simulink model "OUR_BD_FUELCELL"  (R2022b)
settings: Solver=ode1  StartTime=0.0  StopTime=max(cyc_mph(:,1))  FixedStep=1  MaxStep=1  RelTol=1e-3  AbsTol=1e-3
values from neighbouring files (symbols this model uses):
  eta_DC_DC = 1    [main.m]
  fc_pwr_scale = 0.6    [fuelcell_patch.m]
  Ts = 1    [main.m]
undefined symbols (not defined in the file or in its folder): air_cp, amb_tmp, cs_charge_deplete_bool, cs_charge_pwr, cs_fc_init_state, cs_fc_on, cs_hi_soc, cs_lo_soc, cs_max_pwr, cs_max_pwr_fall_rate, cs_max_pwr_rise_rate, cs_min_off_time, cs_min_pwr, ess_on, ex_calc, ex_gas_cp, fc_acc_mass, fc_base_mass, fc_c2i_th_cond, fc_c_init_tmp, fc_cl2h_eff, fc_co_map, fc_co_map_c2h, fc_cold, fc_cold_tmp, fc_cp, fc_eff_scale, fc_emis, fc_emisv, fc_exflow_map, fc_ext_sarea, fc_extmp_map, fc_fuel_den, fc_fuel_lhv, fc_fuel_map, fc_fuel_map_c2h, fc_fuelcell_warmup_bool, fc_h2x_th_cond, fc_h_air_flow, fc_h_cp, fc_h_init_tmp, fc_hc_map, fc_hc_map_c2h, fc_hood_emisv, fc_hood_sarea, fc_i2x_th_cond, fc_i_init_tmp, fc_nox_map, fc_nox_map_c2h, fc_o2_map, fc_on, fc_pm_map, fc_pm_map_c2h, fc_pwr_map, fc_tstat, fc_x_init_tmp, pow, veh_glider_mass
libraries: lib_wheel x2, lib_help x2, lib_transmission x2, lib_outputs x1, lib_controls x1, lib_interactive x1, lib_drive_cycle x1, lib_accessory x1, lib_energy_storage x1, lib_exhaust x1, mpclib x1, lib_electric_machine x1
(part 1 of 2)
settings Model: ModifiedComment=utente -- Tue Jun 25 17:18:19 2024 -- Version 21.0  Creator=mokeefe  LastModifiedBy=William
settings Model: ModifiedHistory=|
  | utente -- Tue Jun 25 17:18:19 2024 -- Version 21.0
  | 
  | mokeefe -- Fri Mar 23 15:51:49 2012 -- Version 1.79
  | Upgrade parameterized links and upgrade file to latest Simulink.
  | 
  | ssprik -- Wed Sep 24 14:55:17 2003 -- Version 1.78
  | 
  | 
  | kharalds -- Tue Jun 10 10:04:01 2003 -- Version 1.77
  | undid the prior change (back to 10000) in Fuel Cell Power System Model/min_cell_voltage & net power gen/algebraic constraint/initial guess
  | 
  | kharalds -- Tue Jun 10 09:48:54 2003 -- Version 1.76
  | in Fuel Cell Power System Model/min_cell_voltage & net power gen/algebraic constraint/Initial guess: changed value from 40000 to 10000.
  | 
  | bjeanner -- Tue Dec 10 15:48:38 2002 -- Version 1.75
  | 
  | 
  | bjeanner -- Tue Dec 10 15:20:32 2002 -- Version 1.74
  | 
  | 
  | bjeanner -- Tue Dec 10 11:52:09 2002 -- Version 1.73
  | 
  | 
  | bjeanner -- Tue Dec 10 11:30:33 2002 -- Version 1.72
  | 
  | 
  | bjeanner -- Tue Dec 10 11:22:18 2002 -- Version 1.71
  | 
  | 
  | bjeanner -- Tue Dec 10 11:18:18 2002 -- Version 1.70
  | 
  | 
  | bjeanner -- Tue Dec 10 10:31:06 2002 -- Version 1.69
  | 
  | 
  | bjeanner -- Tue Dec 10 10:30:27 2002 -- Version 1.68
  | 
  | 
  | bjeanner -- Tue Dec 10 10:23:40 2002 -- Version 1.67
  | 
  | 
  | tmarkel -- Fri Sep 06 14:56:54 2002 -- Version 1.66
  | VT and KTH fuel cell models in place
  | 
  | 
  | tmarkel -- Fri Sep 06 12:17:07 2002 -- Version 1.65
  | akfd
  | 
  | 
  | tmarkel -- Fri Sep 06 11:53:29 2002 -- Version 1.64
  | replaced bad link to altia with link to interactive library block
  | 
  | 
  | tmarkel -- Mon Aug 12 17:09:32 2002 -- Version 1.63
  | trying to get it to see the cinfig sys names
  | 
  | ssprik -- Mon Apr 22 11:29:38 2002 -- Version 1.62
  | 
  | 
  | ssprik -- Mon Apr 22 11:22:32 2002 -- Version 1.61
  | 
  | 
  | ssprik -- Mon Apr 22 11:21:51 2002 -- Version 1.60
  | 
  | 
  | tmarkel -- Sat Apr 20 11:16:25 2002 -- Version 1.59
  | replaced fuel cell linked library model with config system model
  | 
  | 
  | mokeefe -- Thu Apr 18 07:55:48 2002 -- Version 1.58
  | saving the model:
  | o "without the model browser open"
  | o with only top-level screen visible
  | o and with "fit to view" enabled
  | 
  | mokeefe -- Thu Apr 18 07:45:26 2002 -- Version 1.57
  | saving the model:
  | o "without the model browser open"
  | o with only top-level screen visible
  | o and with "fit to view" enabled
settings SolverCC: AutoScaleAbsTol=off  AlgebraicLoopSolver=TrustRegion
settings DataIOCC: SaveFormat=Array  SignalLoggingSaveFormat=ModelDataLogs  SaveOutput=off  SaveTime=off  ReturnWorkspaceOutputs=off
settings OptimizationCC: BooleanDataType=off  ExpressionDepthLimit=2147483647  LifeSpan=inf
settings DebuggingCC: SaveWithParameterizedLinksMsg=none  UnderspecifiedInitializationDetection=Classic  MergeDetectMultiDrivingBlocksExec=none  SignalResolutionControl=TryResolveAllWithWarning  MultiTaskDSMMsg=warning  MultiTaskCondExecSysMsg=none  FcnCallInpInsideContextMsg=warning  UnconnectedInputMsg=warning  UnconnectedOutputMsg=warning  StateNameClashWarn=warning  SFUnexpectedBacktrackingDiag=warning  SFNoUnconditionalDefaultTransitionDiag=warning  SFExecutionAtInitializationDiag=none  SFMachineParentedDataDiag=warning  ArithmeticOperatorsInVariantConditions=warning
settings HardwareCC: ProdBitPerPointer=32  ProdBitPerSizeT=32  ProdBitPerPtrDiffT=32  ProdLargestAtomicFloat=None  ProdIntDivRoundTo=Undefined  ProdEndianess=Unspecified  ProdWordSize=32  ProdHWDeviceType=32-bit Generic  TargetUnknown=on
settings ModelReferenceCC: EnableRefExpFcnMdlSchedulingChecks=on  PropagateSignalLabelsOutOfModel=off
settings SFSimCC: SimUseLocalCustomCode=off  CustomCodeUndefinedFunction=UseInterfaceOnly
settings RTWCC: TemplateMakefile=grt_vc.tmf  RTWUseLocalCustomCode=off
settings CodeAppCC: StateflowObjectComments=on
settings GRTTargetCC: TargetLangStandard=C89/C90 (ANSI)  CombineOutputUpdateFcns=off  GRTInterface=on
settings ConfigComp: CovMetricSettings=dw  CovSaveCumulativeToWorkspaceVar=on  CovSaveSingleToWorkspaceVar=on  CovExternalEMLEnable=off

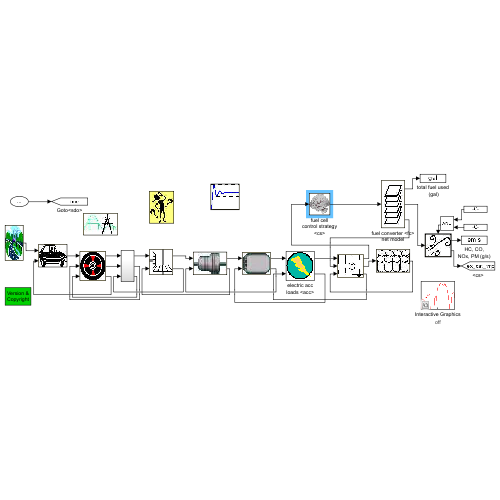
[thumbnail: Simulink's stored preview of the top-level diagram]
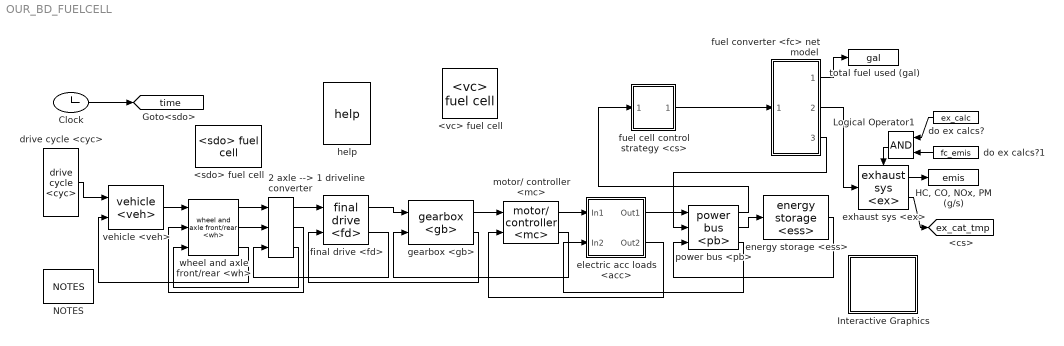
== system OUR_BD_FUELCELL ==
  2 axle --> 1 driveline converter : lib_wheel/2 axle --> 1 driveline converter  SystemSampleTime=-1  VariantActivationTime=update diagram  Latency=0  AutoFrameSizeCalculation=off
  <sdo> fuel cell : lib_outputs/<sdo> fuel cell  SystemSampleTime=-1  VariantActivationTime=update diagram  Latency=0  AutoFrameSizeCalculation=off
  <vc> fuel cell : lib_controls/<vc> fuel cell  SystemSampleTime=-1  VariantActivationTime=update diagram  Latency=0  AutoFrameSizeCalculation=off
      link override config traction control: BlockChoice=traction control 2 axle
  Clock : Clock
  "HC, CO, NOx, PM (g/s)" : ToWorkspace  VariableName=emis
  Interactive Graphics : Subsystem  BlockChoice=off
      link override off/Live Inputs/veh/roll res interactive: BlockChoice=roll res force req (N)
      settings: AttributesFormatString=%<BlockChoice>  TemplateBlock=lib_interactive/Interactive Graphics  MemberBlocks=off,on
  Logical Operator1 : Logic
  NOTES : lib_help/NOTES  SystemSampleTime=-1  VariantActivationTime=update diagram  Latency=0  AutoFrameSizeCalculation=off
  do ex calcs? : Constant  Value=ex_calc
  do ex calcs?1 : Constant  Value=fc_emis
  drive cycle <cyc> : lib_drive_cycle/drive cycle <cyc>  SystemSampleTime=-1  VariantActivationTime=update diagram  Latency=0  AutoFrameSizeCalculation=off
  electric acc loads <acc> : Subsystem
      mask Display: image(imread('bdi_acc_elec.bmp'))
  energy storage <ess> : lib_energy_storage/energy storage <ess>  SystemSampleTime=-1  VariantActivationTime=update diagram  Latency=0  AutoFrameSizeCalculation=off
      link override ess config: BlockChoice=energy storage <ess>
  exhaust sys <ex> : lib_exhaust/exhaust sys <ex>  SystemSampleTime=-1  VariantActivationTime=update diagram  Latency=0  AutoFrameSizeCalculation=off
  final drive <fd> : lib_transmission/final drive <fd>  SystemSampleTime=-1  VariantActivationTime=update diagram  Latency=0  AutoFrameSizeCalculation=off
  fuel cell control strategy <cs> : Subsystem  AncestorBlock=|
      | lib_controls/fuel cell
      | control strategy
      | <cs>
      settings: LibrarySourceBlock=|
      | lib_controls/fuel cell
      | control strategy
      | <cs>
      mask Display: image(imread('bdi_cs.jpg'))
  fuel converter <fc> net model : Subsystem  VariantControl=fuel converter <fc> net model
      mask Display: image(imread('bdi_fuelcell.jpg'))
  gearbox <gb> : lib_transmission/gearbox <gb>  SystemSampleTime=-1  VariantActivationTime=update diagram  Latency=0  AutoFrameSizeCalculation=off
  help : lib_help/help  SystemSampleTime=-1  VariantActivationTime=update diagram  Latency=0  AutoFrameSizeCalculation=off
  motor/ controller <mc> : lib_electric_machine/motor// controller <mc>  SystemSampleTime=-1  VariantActivationTime=update diagram  Latency=0  AutoFrameSizeCalculation=off
  power bus <pb> : lib_power_bus/power bus <pb>  SystemSampleTime=-1  VariantActivationTime=update diagram  Latency=0  AutoFrameSizeCalculation=off
  total fuel used (gal) : ToWorkspace  VariableName=gal
  vehicle <veh> : lib_vehicle/vehicle <veh>  SystemSampleTime=-1  VariantActivationTime=update diagram  Latency=0  AutoFrameSizeCalculation=off
      link override record achieved force outputs/rolling resistance force: BlockChoice=force req'd to overcome rolling resistance (N)
      link override rolling resistance force: BlockChoice=force req'd to overcome rolling resistance (N)
      link override vehicle speed: BlockChoice=vehicle speed (m/s)
  wheel and axle front/rear <wh> : lib_wheel/wheel and axle  front//rear <wh>  SystemSampleTime=-1  VariantActivationTime=update diagram  Latency=0  AutoFrameSizeCalculation=off
  tag scope: ex_cat_tmp=global, time=global
  wires:
  final drive <fd>/2 -> 2 axle --> 1 driveline converter/3
  2 axle --> 1 driveline converter/1 -> final drive <fd>/1
  wheel and axle front/rear <wh>/3 -> vehicle <veh>/2
  final drive <fd>/1 -> gearbox <gb>/1
  drive cycle <cyc>/1 -> vehicle <veh>/1
  Clock/1 -> [time]
  energy storage <ess>/1 -> power bus <pb>/3
  power bus <pb>/2 -> energy storage <ess>/1
  motor/ controller <mc>/2 -> gearbox <gb>/2
  gearbox <gb>/1 -> motor/ controller <mc>/1
  gearbox <gb>/2 -> final drive <fd>/2
  power bus <pb>/1 -> fuel cell control strategy <cs>/1(power req'd by bus (W)1)
  fuel cell control strategy <cs>/1(engine pwr (W)1) -> fuel converter <fc> net model/1(pwr req'd at fc output (W))
  fuel converter <fc> net model/2(EO emis info) -> exhaust sys <ex>/1
  fuel converter <fc> net model/1(fuel use) -> total fuel used (gal)/1
  do ex calcs?/1 -> Logical Operator1/1
  exhaust sys <ex>/1 -> "HC, CO, NOx, PM (g/s)"/1
  Logical Operator1/1 -> exhaust sys <ex>/Enable
  do ex calcs?1/1 -> Logical Operator1/2
  fuel converter <fc> net model/3(pwr avail. to driveline (W)) -> power bus <pb>/2
  exhaust sys <ex>/2 -> [ex_cat_tmp]
  motor/ controller <mc>/1 -> electric acc loads <acc>/1(In1)
  electric acc loads <acc>/1(Out1) -> power bus <pb>/1
  power bus <pb>/3 -> electric acc loads <acc>/2(In2)
  electric acc loads <acc>/2(Out2) -> motor/ controller <mc>/2
  wheel and axle front/rear <wh>/1 -> 2 axle --> 1 driveline converter/1
  wheel and axle front/rear <wh>/2 -> 2 axle --> 1 driveline converter/2
  2 axle --> 1 driveline converter/2 -> wheel and axle front/rear <wh>/2
  2 axle --> 1 driveline converter/3 -> wheel and axle front/rear <wh>/3
  vehicle <veh>/1 -> wheel and axle front/rear <wh>/1

== system OUR_BD_FUELCELL/Interactive Graphics ==
  off : lib_interactive/off  Tag=Altia_off  SystemSampleTime=-1  VariantActivationTime=update diagram  Latency=0  AutoFrameSizeCalculation=off

== system OUR_BD_FUELCELL/electric acc loads <acc> ==
  note: from vc
  In1 : Inport
  In2 : Inport  Port=2
  Electrical Accessory Loads v2 <acc> : lib_accessory/Electrical Accessory Loads v2 <acc>  load_on=1
      link override backward model/electrical accessories (W): BlockChoice=Electrical Accessories: Time Variable
  Out1 : Outport
  Out2 : Outport  Port=2
  wires:
  In1/1 -> Electrical Accessory Loads v2 <acc>/1
  In2/1 -> Electrical Accessory Loads v2 <acc>/2
  Electrical Accessory Loads v2 <acc>/1 -> Out1/1
  Electrical Accessory Loads v2 <acc>/2 -> Out2/1
  [key_on] -> Electrical Accessory Loads v2 <acc>/3

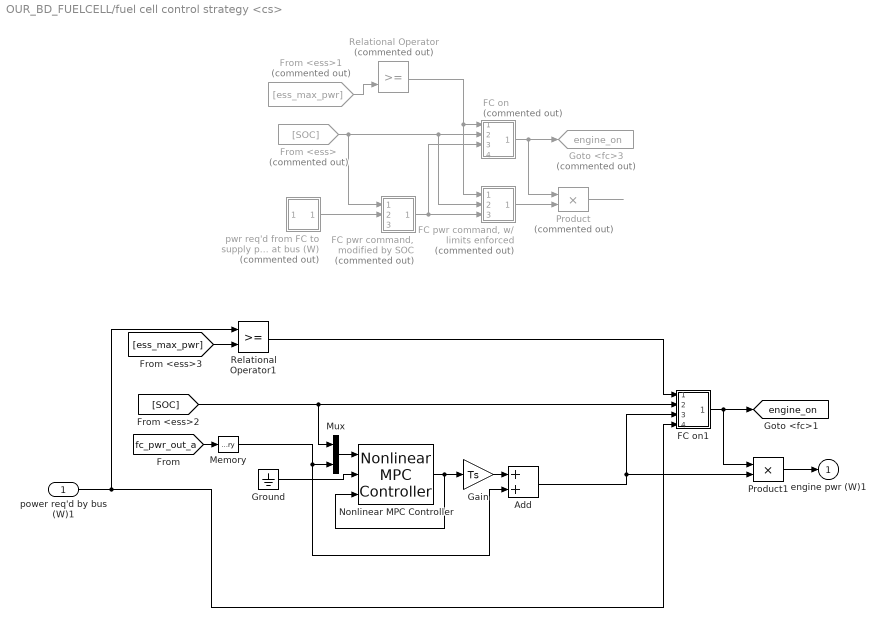
== system OUR_BD_FUELCELL/fuel cell control strategy <cs> ==
  power req'd by bus (W)1 : Inport
  Add : Sum
  FC on : Subsystem  Commented=on
  FC on1 : Subsystem
  "FC pwr command, modified by SOC" : Subsystem  Commented=on
  "FC pwr command, w/ limits enforced" : Subsystem  Commented=on
  From <ess> : From  Commented=on  GotoTag=SOC
      settings: CloseFcn=tagdialog Close
  From <ess>1 : From  Commented=on  GotoTag=ess_max_pwr
      settings: CloseFcn=tagdialog Close
  Gain : Gain  Gain=Ts
  Goto <fc>3 : Goto  Commented=on  GotoTag=engine_on  TagVisibility=global
  Ground : Ground
  Memory : Memory
  Mux : Mux  Inputs=2
  Nonlinear MPC Controller : mpclib/Nonlinear MPC Controller  nlmpcobj=nlobj  UseObjectTs=on  UseMEX=off  md_enabled=off  mvtarget_enabled=off  param_enabled=off  cost_enabled=off  mvseq_enabled=off  stateseq_enabled=off  ovseq_enabled=off  slack_enabled=off  status_enabled=off  ov_min=off  ov_max=off  mv_min=off  mv_max=off  mvrate_min=off  mvrate_max=off  state_min=off  state_max=off  ov_weight=off  mv_weight=off  mvrate_weight=off  ecr_weight=off  nlp_initialize=off
  Product : Product  Commented=on  InputSameDT=on  RndMeth=Zero  SaturateOnIntegerOverflow=on  OutDataTypeStr=Inherit: Same as first input
  Product1 : Product  InputSameDT=on  RndMeth=Zero  SaturateOnIntegerOverflow=on  OutDataTypeStr=Inherit: Same as first input
  Relational Operator : RelationalOperator  Commented=on
  Relational Operator1 : RelationalOperator
  pwr req'd from FC to supply pwr req'd at bus (W) : Subsystem  Commented=on
  engine pwr (W)1 : Outport  InitialOutput=0
  tag scope: engine_on=global
  wires:
  ? -> FC on/4(bus pwr req), "FC pwr command, modified by SOC"/3(pwr req'd at bus (W)), Relational Operator/1, pwr req'd from FC to supply pwr req'd at bus (W)/1(power req'd by bus (W))
  From <ess>1/1 -> Relational Operator/2
  Product/1 -> ?
  pwr req'd from FC to supply pwr req'd at bus (W)/1(pwr req'd of FC (W)) -> "FC pwr command, modified by SOC"/2(raw pwr command (W))
  "FC pwr command, w/ limits enforced"/1(limited FC pwr command (W)) -> Product/2
  Relational Operator/1 -> FC on/1(ess max pwr would be insufficient), "FC pwr command, w/ limits enforced"/1(ess max pwr would be insufficient)
  From <ess>/1 -> "FC pwr command, modified by SOC"/1(SOC), FC on/2(SOC), "FC pwr command, w/ limits enforced"/2(SOC)
  "FC pwr command, modified by SOC"/1(pwr command modifed for SOC (W)) -> "FC pwr command, w/ limits enforced"/3(FC pwr command), FC on/3(FC pwr command)
  FC on/1(FC on) -> Goto <fc>3/1, Product/1
  [SOC] -> Mux/1, FC on1/2(SOC)
  Relational Operator1/1 -> FC on1/1(ess max pwr would be insufficient)
  power req'd by bus (W)1/1 -> FC on1/4(bus pwr req), Relational Operator1/1
  FC on1/1(FC on) -> [engine_on], Product1/1
  Add/1 -> FC on1/3(FC pwr command), Product1/2
  Product1/1 -> engine pwr (W)1/1
  [ess_max_pwr] -> Relational Operator1/2
  Nonlinear MPC Controller/1 -> Nonlinear MPC Controller/3, Gain/1
  Gain/1 -> Add/1
  [fc_pwr_out_a] -> Memory/1
  Memory/1 -> Mux/2, Add/2
  Mux/1 -> Nonlinear MPC Controller/1
  Ground/1 -> Nonlinear MPC Controller/2

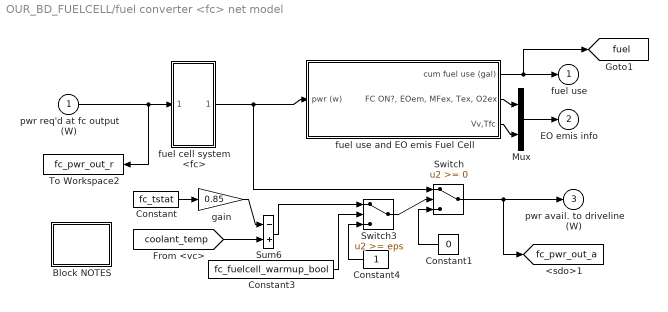
== system OUR_BD_FUELCELL/fuel converter <fc> net model ==
  pwr req'd at fc output (W) : Inport
  Block NOTES : Subsystem
      mask Display: disp('Block\nNOTES')
  Constant : Constant  Value=fc_tstat
  Constant1 : Constant  Value=0
  Constant3 : Constant  Value=fc_fuelcell_warmup_bool
  Constant4 : Constant
  Mux : Mux  Inputs=2
  Sum6 : Sum  Inputs=-+  InputSameDT=on  SaturateOnIntegerOverflow=on  OutDataTypeStr=Inherit: Same as first input
  Switch : Switch
  Switch3 : Switch  Threshold=eps
  To Workspace2 : ToWorkspace  VariableName=fc_pwr_out_r  SampleTime=-1
  fuel cell system <fc> : Subsystem
  fuel use and EO emis Fuel Cell : Subsystem
  gain : Gain  Gain=0.85  SaturateOnIntegerOverflow=on  OutDataTypeStr=Inherit: Same as input  ParamDataTypeStr=Inherit: Same as input
  fuel use : Outport  InitialOutput=0
  EO emis info : Outport  Port=2  InitialOutput=0
  pwr avail. to driveline (W) : Outport  Port=3  InitialOutput=0
  tag scope: fc_pwr_out_a=global, fuel=global
  wires:
  fuel use and EO emis Fuel Cell/1(cum fuel use (gal)) -> [fuel], fuel use/1
  [coolant_temp] -> Sum6/2
  gain/1 -> Sum6/1
  Constant/1 -> gain/1
  Switch/1 -> [fc_pwr_out_a], pwr avail. to driveline (W)/1
  Switch3/1 -> Switch/2
  Sum6/1 -> Switch3/1
  Constant4/1 -> Switch3/3
  Constant3/1 -> Switch3/2
  Constant1/1 -> Switch/3
  pwr req'd at fc output (W)/1 -> fuel cell system <fc>/1(pwr req (W)), To Workspace2/1
  fuel cell system <fc>/1(power available (W) 1x1) -> Switch/1, fuel use and EO emis Fuel Cell/1(pwr (w))
  fuel use and EO emis Fuel Cell/3(Vv,Tfc) -> Mux/2
  fuel use and EO emis Fuel Cell/2("FC ON?, EOem, MFex, Tex, O2ex") -> Mux/1
  Mux/1 -> EO emis info/1

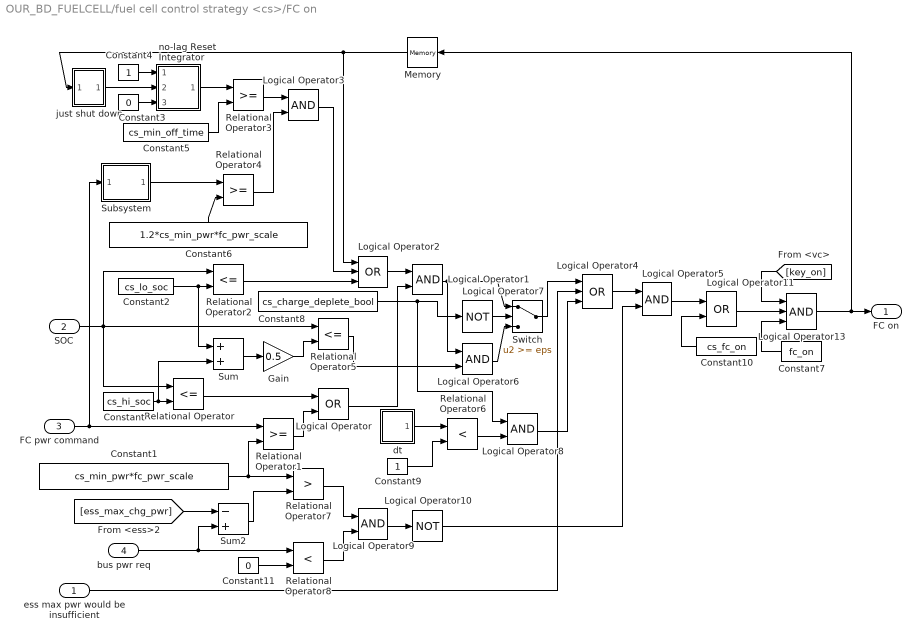
== system OUR_BD_FUELCELL/fuel cell control strategy <cs>/FC on ==
  ess max pwr would be insufficient : Inport
  SOC : Inport  Port=2
  FC pwr command : Inport  Port=3
  bus pwr req : Inport  Port=4
  Constant : Constant  Value=cs_hi_soc
  Constant1 : Constant  Value=cs_min_pwr*fc_pwr_scale
  Constant10 : Constant  Value=cs_fc_on
  Constant11 : Constant  Value=0
  Constant2 : Constant  Value=cs_lo_soc
  Constant3 : Constant  Value=0
  Constant4 : Constant
  Constant5 : Constant  Value=cs_min_off_time
  Constant6 : Constant  Value=1.2*cs_min_pwr*fc_pwr_scale
  Constant7 : Constant  Value=fc_on
  Constant8 : Constant  Value=cs_charge_deplete_bool
  Constant9 : Constant
  Gain : Gain  Gain=0.5  SaturateOnIntegerOverflow=on  OutDataTypeStr=Inherit: Same as input  ParamDataTypeStr=Inherit: Same as input
  Logical Operator : Logic  Operator=OR
  Logical Operator{1,3,5..6,8..9} (6 alike) : Logic
  Logical Operator10 : Logic  Operator=NOT
  Logical Operator11 : Logic  Operator=OR
  Logical Operator13 : Logic  Inputs=3
  Logical Operator2 : Logic  Operator=OR  Inputs=3
  Logical Operator4 : Logic  Operator=OR  Inputs=3
  Logical Operator7 : Logic  Operator=NOT  Inputs=1
  Memory : Memory  InitialCondition=cs_fc_init_state
  Relational Operator : RelationalOperator  Operator=<=
  Relational Operator1 : RelationalOperator
  Relational Operator2 : RelationalOperator  Operator=<=
  Relational Operator3 : RelationalOperator
  Relational Operator4 : RelationalOperator
  Relational Operator5 : RelationalOperator  Operator=<=
  Relational Operator6 : RelationalOperator  Operator=<
  Relational Operator7 : RelationalOperator  Operator=>
  Relational Operator8 : RelationalOperator  Operator=<
  Subsystem : Subsystem  mask(Running Average){n=5}
      mask prompts: n "Averaging Time (s)"
      mask help: Running Average
      mask Help: Output is the average of the last (Averaging Time) seconds of input.
      mask Display: disp('Running\nAverage')
  Sum : Sum  InputSameDT=on  SaturateOnIntegerOverflow=on  OutDataTypeStr=Inherit: Same as first input
  Sum2 : Sum  Inputs=-+  InputSameDT=on  SaturateOnIntegerOverflow=on  OutDataTypeStr=Inherit: Same as first input
  Switch : Switch  Threshold=eps
  dt : Subsystem
  just shut down : Subsystem
  no-lag Reset Integrator : Subsystem  mask(No-lag Reset Integrator){initval=0}
      mask prompts: initval "Initial Value"
      mask help: No-lag Reset Integrator
      mask Help: Integrates first input using Euler technique.\nAt the time step that input 2 <> zero,\noutput is reset to input 3.
      mask Display: disp('1/s\nw/ reset\nno lag')
  FC on : Outport
  wires:
  Relational Operator6/1 -> Logical Operator8/2
  Constant9/1 -> Relational Operator6/2
  dt/1(out_1) -> Relational Operator6/1
  Logical Operator8/1 -> Logical Operator4/3
  Constant8/1 -> Logical Operator8/1, Logical Operator7/1
  Switch/1 -> Logical Operator4/1
  Logical Operator1/1 -> Logical Operator6/1, Switch/1
  Logical Operator6/1 -> Switch/3
  Logical Operator7/1 -> Switch/2
  Gain/1 -> Relational Operator5/2
  Sum/1 -> Gain/1
  Constant/1 -> Sum/2, Relational Operator/2
  Constant2/1 -> Sum/1, Relational Operator2/2
  Memory/1 -> just shut down/1(state), Logical Operator2/1
  Constant5/1 -> Relational Operator3/2
  Relational Operator3/1 -> Logical Operator3/1
  no-lag Reset Integrator/1(out_1) -> Relational Operator3/1
  just shut down/1(trigger) -> no-lag Reset Integrator/2(in_2)
  Constant3/1 -> no-lag Reset Integrator/3(in_3)
  Constant4/1 -> no-lag Reset Integrator/1(in_1)
  Constant6/1 -> Relational Operator4/2
  Relational Operator4/1 -> Logical Operator3/2
  Subsystem/1(out_1) -> Relational Operator4/1
  Logical Operator3/1 -> Logical Operator2/2
  Logical Operator2/1 -> Logical Operator1/1
  SOC/1 -> Relational Operator5/1, Relational Operator/1, Relational Operator2/1
  Relational Operator1/1 -> Logical Operator/2
  FC pwr command/1 -> Relational Operator1/1, Subsystem/1(in_1)
  ess max pwr would be insufficient/1 -> Logical Operator4/2
  Relational Operator5/1 -> Logical Operator6/2
  Relational Operator2/1 -> Logical Operator2/3
  Relational Operator/1 -> Logical Operator/1
  Constant11/1 -> Relational Operator8/2
  [ess_max_chg_pwr] -> Sum2/1
  bus pwr req/1 -> Relational Operator8/1, Sum2/2
  Sum2/1 -> Relational Operator7/2
  Logical Operator/1 -> Logical Operator1/2
  Logical Operator9/1 -> Logical Operator10/1
  Logical Operator10/1 -> Logical Operator5/2
  Relational Operator7/1 -> Logical Operator9/1
  Relational Operator8/1 -> Logical Operator9/2
  Constant1/1 -> Relational Operator1/2, Relational Operator7/1
  Logical Operator5/1 -> Logical Operator11/1
  Constant10/1 -> Logical Operator11/2
  Logical Operator4/1 -> Logical Operator5/1
  Logical Operator11/1 -> Logical Operator13/2
  [key_on] -> Logical Operator13/1
  Constant7/1 -> Logical Operator13/3
  Logical Operator13/1 -> FC on/1, Memory/1

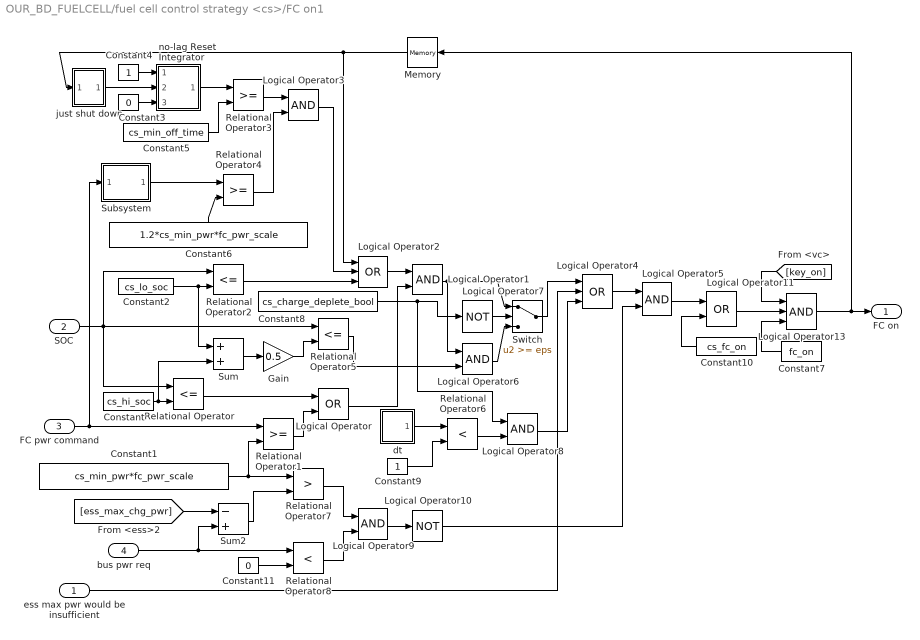
== system OUR_BD_FUELCELL/fuel cell control strategy <cs>/FC on1 ==
  ess max pwr would be insufficient : Inport
  SOC : Inport  Port=2
  FC pwr command : Inport  Port=3
  bus pwr req : Inport  Port=4
  Constant : Constant  Value=cs_hi_soc
  Constant1 : Constant  Value=cs_min_pwr*fc_pwr_scale
  Constant10 : Constant  Value=cs_fc_on
  Constant11 : Constant  Value=0
  Constant2 : Constant  Value=cs_lo_soc
  Constant3 : Constant  Value=0
  Constant4 : Constant
  Constant5 : Constant  Value=cs_min_off_time
  Constant6 : Constant  Value=1.2*cs_min_pwr*fc_pwr_scale
  Constant7 : Constant  Value=fc_on
  Constant8 : Constant  Value=cs_charge_deplete_bool
  Constant9 : Constant
  Gain : Gain  Gain=0.5  SaturateOnIntegerOverflow=on  OutDataTypeStr=Inherit: Same as input  ParamDataTypeStr=Inherit: Same as input
  Logical Operator : Logic  Operator=OR
  Logical Operator{1,3,5..6,8..9} (6 alike) : Logic
  Logical Operator10 : Logic  Operator=NOT
  Logical Operator11 : Logic  Operator=OR
  Logical Operator13 : Logic  Inputs=3
  Logical Operator2 : Logic  Operator=OR  Inputs=3
  Logical Operator4 : Logic  Operator=OR  Inputs=3
  Logical Operator7 : Logic  Operator=NOT  Inputs=1
  Memory : Memory  InitialCondition=cs_fc_init_state
  Relational Operator : RelationalOperator  Operator=<=
  Relational Operator1 : RelationalOperator
  Relational Operator2 : RelationalOperator  Operator=<=
  Relational Operator3 : RelationalOperator
  Relational Operator4 : RelationalOperator
  Relational Operator5 : RelationalOperator  Operator=<=
  Relational Operator6 : RelationalOperator  Operator=<
  Relational Operator7 : RelationalOperator  Operator=>
  Relational Operator8 : RelationalOperator  Operator=<
  Subsystem : Subsystem  mask(Running Average){n=5}
      mask prompts: n "Averaging Time (s)"
      mask help: Running Average
      mask Help: Output is the average of the last (Averaging Time) seconds of input.
      mask Display: disp('Running\nAverage')
  Sum : Sum  InputSameDT=on  SaturateOnIntegerOverflow=on  OutDataTypeStr=Inherit: Same as first input
  Sum2 : Sum  Inputs=-+  InputSameDT=on  SaturateOnIntegerOverflow=on  OutDataTypeStr=Inherit: Same as first input
  Switch : Switch  Threshold=eps
  dt : Subsystem
  just shut down : Subsystem
  no-lag Reset Integrator : Subsystem  mask(No-lag Reset Integrator){initval=0}
      mask prompts: initval "Initial Value"
      mask help: No-lag Reset Integrator
      mask Help: Integrates first input using Euler technique.\nAt the time step that input 2 <> zero,\noutput is reset to input 3.
      mask Display: disp('1/s\nw/ reset\nno lag')
  FC on : Outport
  wires:
  Relational Operator6/1 -> Logical Operator8/2
  Constant9/1 -> Relational Operator6/2
  dt/1(out_1) -> Relational Operator6/1
  Logical Operator8/1 -> Logical Operator4/3
  Constant8/1 -> Logical Operator8/1, Logical Operator7/1
  Switch/1 -> Logical Operator4/1
  Logical Operator1/1 -> Logical Operator6/1, Switch/1
  Logical Operator6/1 -> Switch/3
  Logical Operator7/1 -> Switch/2
  Gain/1 -> Relational Operator5/2
  Sum/1 -> Gain/1
  Constant/1 -> Sum/2, Relational Operator/2
  Constant2/1 -> Sum/1, Relational Operator2/2
  Memory/1 -> just shut down/1(state), Logical Operator2/1
  Constant5/1 -> Relational Operator3/2
  Relational Operator3/1 -> Logical Operator3/1
  no-lag Reset Integrator/1(out_1) -> Relational Operator3/1
  just shut down/1(trigger) -> no-lag Reset Integrator/2(in_2)
  Constant3/1 -> no-lag Reset Integrator/3(in_3)
  Constant4/1 -> no-lag Reset Integrator/1(in_1)
  Constant6/1 -> Relational Operator4/2
  Relational Operator4/1 -> Logical Operator3/2
  Subsystem/1(out_1) -> Relational Operator4/1
  Logical Operator3/1 -> Logical Operator2/2
  Logical Operator2/1 -> Logical Operator1/1
  SOC/1 -> Relational Operator5/1, Relational Operator/1, Relational Operator2/1
  Relational Operator1/1 -> Logical Operator/2
  FC pwr command/1 -> Relational Operator1/1, Subsystem/1(in_1)
  ess max pwr would be insufficient/1 -> Logical Operator4/2
  Relational Operator5/1 -> Logical Operator6/2
  Relational Operator2/1 -> Logical Operator2/3
  Relational Operator/1 -> Logical Operator/1
  Constant11/1 -> Relational Operator8/2
  [ess_max_chg_pwr] -> Sum2/1
  bus pwr req/1 -> Relational Operator8/1, Sum2/2
  Sum2/1 -> Relational Operator7/2
  Logical Operator/1 -> Logical Operator1/2
  Logical Operator9/1 -> Logical Operator10/1
  Logical Operator10/1 -> Logical Operator5/2
  Relational Operator7/1 -> Logical Operator9/1
  Relational Operator8/1 -> Logical Operator9/2
  Constant1/1 -> Relational Operator1/2, Relational Operator7/1
  Logical Operator5/1 -> Logical Operator11/1
  Constant10/1 -> Logical Operator11/2
  Logical Operator4/1 -> Logical Operator5/1
  Logical Operator11/1 -> Logical Operator13/2
  [key_on] -> Logical Operator13/1
  Constant7/1 -> Logical Operator13/3
  Logical Operator13/1 -> FC on/1, Memory/1

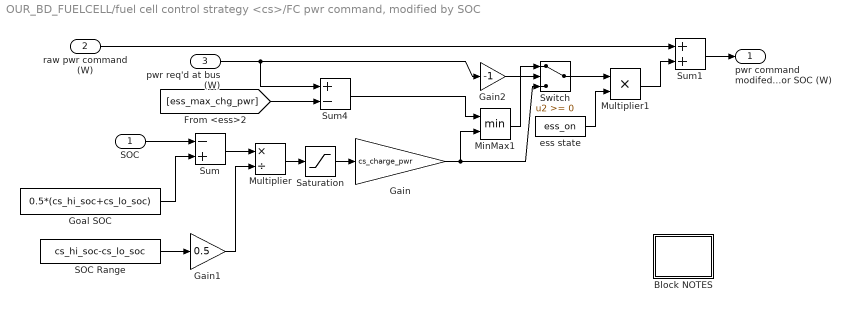
== system OUR_BD_FUELCELL/fuel cell control strategy <cs>/FC pwr command, modified by SOC ==
  SOC : Inport
  raw pwr command (W) : Inport  Port=2
  pwr req'd at bus (W) : Inport  Port=3
  Block NOTES : Subsystem
      mask Display: disp('Block\nNOTES')
  Gain : Gain  Gain=cs_charge_pwr  SaturateOnIntegerOverflow=on  OutDataTypeStr=Inherit: Same as input  ParamDataTypeStr=Inherit: Same as input
  Gain1 : Gain  Gain=0.5  SaturateOnIntegerOverflow=on  OutDataTypeStr=Inherit: Same as input  ParamDataTypeStr=Inherit: Same as input
  Gain2 : Gain  Gain=-1  SaturateOnIntegerOverflow=on  OutDataTypeStr=Inherit: Same as input  ParamDataTypeStr=Inherit: Same as input
  Goal SOC : Constant  Value=0.5*(cs_hi_soc+cs_lo_soc)
  MinMax1 : MinMax  Inputs=2  InputSameDT=on  SaturateOnIntegerOverflow=on
  Multiplier : Product  Inputs=*/  InputSameDT=on  RndMeth=Zero  SaturateOnIntegerOverflow=on  OutDataTypeStr=Inherit: Same as first input
  Multiplier1 : Product  InputSameDT=on  RndMeth=Zero  SaturateOnIntegerOverflow=on  OutDataTypeStr=Inherit: Same as first input
  SOC Range : Constant  Value=cs_hi_soc-cs_lo_soc
  Saturation : Saturate  UpperLimit=1  LowerLimit=-1
  Sum : Sum  Inputs=-+  InputSameDT=on  SaturateOnIntegerOverflow=on  OutDataTypeStr=Inherit: Same as first input
  Sum1 : Sum  InputSameDT=on  SaturateOnIntegerOverflow=on  OutDataTypeStr=Inherit: Same as first input
  Sum4 : Sum  Inputs=+-  InputSameDT=on  SaturateOnIntegerOverflow=on  OutDataTypeStr=Inherit: Same as first input
  Switch : Switch
  ess state : Constant  Value=ess_on
  pwr command modifed for SOC (W) : Outport
  wires:
  SOC/1 -> Sum/1
  Goal SOC/1 -> Sum/2
  SOC Range/1 -> Gain1/1
  Multiplier/1 -> Saturation/1
  Sum/1 -> Multiplier/1
  Saturation/1 -> Gain/1
  Gain1/1 -> Multiplier/2
  MinMax1/1 -> Switch/1
  Gain/1 -> MinMax1/2, Switch/3
  Gain2/1 -> Switch/2
  raw pwr command (W)/1 -> Sum1/1
  pwr req'd at bus (W)/1 -> Sum4/1, Gain2/1
  [ess_max_chg_pwr] -> Sum4/2
  Sum4/1 -> MinMax1/1
  Sum1/1 -> pwr command modifed for SOC (W)/1
  ess state/1 -> Multiplier1/2
  Switch/1 -> Multiplier1/1
  Multiplier1/1 -> Sum1/2

== system OUR_BD_FUELCELL/fuel cell control strategy <cs>/FC pwr command, w// limits enforced ==
  ess max pwr would be insufficient : Inport
  SOC : Inport  Port=2
  FC pwr command : Inport  Port=3
  Constant : Constant  Value=cs_min_pwr*fc_pwr_scale
  Constant1 : Constant  Value=cs_lo_soc
  Constant2 : Constant  Value=cs_max_pwr*fc_pwr_scale
  Logical Operator : Logic  Inputs=3
  Logical Operator1 : Logic  Operator=NOT  Inputs=1
  MinMax : MinMax  Function=max  Inputs=2  InputSameDT=on  SaturateOnIntegerOverflow=on
  MinMax1 : MinMax  Inputs=2  InputSameDT=on  SaturateOnIntegerOverflow=on
  Rate Limiter : RateLimiter  RisingSlewLimit=cs_max_pwr_rise_rate*fc_pwr_scale  FallingSlewLimit=cs_max_pwr_fall_rate*fc_pwr_scale
  Relational Operator : RelationalOperator
  Switch : Switch  Threshold=eps
  ess state : Constant  Value=ess_on
  limited FC pwr command (W) : Outport
  wires:
  ess max pwr would be insufficient/1 -> Logical Operator1/1
  Logical Operator1/1 -> Logical Operator/1
  Relational Operator/1 -> Logical Operator/2
  SOC/1 -> Relational Operator/1
  Logical Operator/1 -> Switch/2
  Constant1/1 -> Relational Operator/2
  Rate Limiter/1 -> limited FC pwr command (W)/1
  Switch/1 -> Rate Limiter/1
  MinMax/1 -> Switch/3, MinMax1/2
  MinMax1/1 -> Switch/1
  Constant2/1 -> MinMax1/1
  Constant/1 -> MinMax/2
  FC pwr command/1 -> MinMax/1
  ess state/1 -> Logical Operator/3

== system OUR_BD_FUELCELL/fuel cell control strategy <cs>/pwr req'd from FC to supply pwr req'd at bus (W) ==
  power req'd by bus (W) : Inport
  Constant2 : Constant  Value=0
  Constant3 : Constant  Value=0
  Relational Operator : RelationalOperator  Operator=>
  Switch : Switch  Threshold=eps
  pwr req'd of FC (W) : Outport
  wires:
  power req'd by bus (W)/1 -> Relational Operator/1, Switch/1
  Constant2/1 -> Relational Operator/2
  Constant3/1 -> Switch/3
  Relational Operator/1 -> Switch/2
  Switch/1 -> pwr req'd of FC (W)/1

== system OUR_BD_FUELCELL/fuel converter <fc> net model/Block NOTES ==
  note: This block models the internal combustion engine, and includes inertia effects,
      | performance limits, accessory loads, and temperature transient effects on fuel
      | use, engine-out emissions, and catalyst efficiency.  There are 'leads' to the
      | engine controller here, which controller determines whether the engine is on.

== system OUR_BD_FUELCELL/fuel converter <fc> net model/fuel cell system <fc> ==
  pwr req (W) : Inport
  Block NOTES : Subsystem
      mask Display: disp('Block\nNOTES')
  pwr vs. eff fuel cell model : Subsystem  TreatAsAtomicUnit=on
  power available (W) 1x1 : Outport  InitialOutput=0
  wires:
  pwr vs. eff fuel cell model/1(net pwr avail (W)) -> power available (W) 1x1/1
  [engine_on] -> pwr vs. eff fuel cell model/Enable
  pwr req (W)/1 -> pwr vs. eff fuel cell model/1(net pwr req (W))

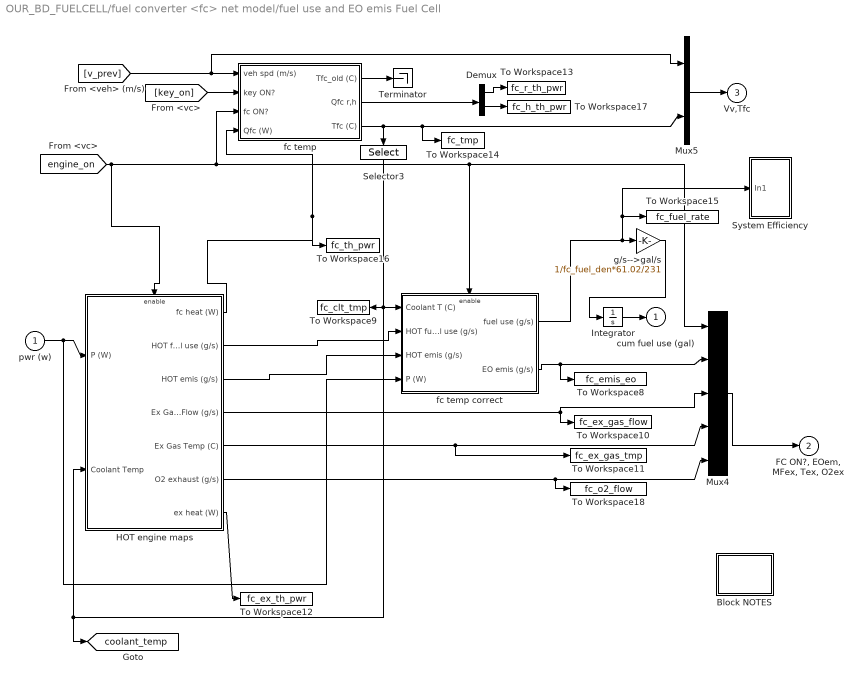
== system OUR_BD_FUELCELL/fuel converter <fc> net model/fuel use and EO emis Fuel Cell ==
  pwr (w) : Inport
  Block NOTES : Subsystem
      mask Display: disp('Block\nNOTES')
  Demux : Demux  Outputs=2
      settings: DisplayOption=none
  "HOT engine maps " : Subsystem  TreatAsAtomicUnit=on
  Integrator : Integrator
  Mux4 : Mux  Inputs=[1 4 1 1 1]
  Mux5 : Mux  Inputs=[1 4 ]
  Selector3 : Selector  InputPortWidth=4  IndexOptions=Index vector (dialog)  Indices=2  OutputSizes=1
  System Efficiency : Subsystem
  Terminator : Terminator
  To Workspace10 : ToWorkspace  VariableName=fc_ex_gas_flow  SampleTime=-1
  To Workspace11 : ToWorkspace  VariableName=fc_ex_gas_tmp  SampleTime=-1
  To Workspace12 : ToWorkspace  VariableName=fc_ex_th_pwr  SampleTime=-1
  To Workspace13 : ToWorkspace  VariableName=fc_r_th_pwr  SampleTime=-1
  To Workspace14 : ToWorkspace  VariableName=fc_tmp  SampleTime=-1
  To Workspace15 : ToWorkspace  VariableName=fc_fuel_rate  SampleTime=-1
  To Workspace16 : ToWorkspace  VariableName=fc_th_pwr  SampleTime=-1
  To Workspace17 : ToWorkspace  VariableName=fc_h_th_pwr  SampleTime=-1
  To Workspace18 : ToWorkspace  VariableName=fc_o2_flow  SampleTime=-1
  To Workspace8 : ToWorkspace  VariableName=fc_emis_eo  SampleTime=-1
  To Workspace9 : ToWorkspace  VariableName=fc_clt_tmp  SampleTime=-1
  fc temp : Subsystem
  fc temp correct : Subsystem  TreatAsAtomicUnit=on
  g/s-->gal/s : Gain  Gain=1/fc_fuel_den*61.02/231  SaturateOnIntegerOverflow=on  OutDataTypeStr=Inherit: Same as input  ParamDataTypeStr=Inherit: Same as input
  cum fuel use (gal) : Outport  InitialOutput=0
  "FC ON?, EOem, MFex, Tex, O2ex" : Outport  Port=2  InitialOutput=0
  Vv,Tfc : Outport  Port=3  InitialOutput=0
  tag scope: coolant_temp=global
  wires:
  "HOT engine maps "/1(fc heat (W)) -> To Workspace16/1, fc temp/4(Qfc (W))
  pwr (w)/1 -> fc temp correct/4(P (W)), "HOT engine maps "/1(P (W))
  "HOT engine maps "/3(HOT emis (g/s)) -> fc temp correct/3(HOT emis (g/s))
  Mux5/1 -> Vv,Tfc/1
  [v_prev] -> Mux5/1, fc temp/1(veh spd (m/s))
  fc temp/3(Tfc (C)) -> Selector3/1, To Workspace14/1, Mux5/2
  fc temp/1(Tfc_old (C)) -> Terminator/1
  fc temp/2(Qfc r,h) -> Demux/1
  Demux/1 -> To Workspace13/1
  Demux/2 -> To Workspace17/1
  [key_on] -> fc temp/2(key ON?)
  "HOT engine maps "/5(Ex Gas Temp (C)) -> To Workspace11/1, Mux4/4
  "HOT engine maps "/4(Ex Gas Flow (g/s)) -> Mux4/3, To Workspace10/1
  Mux4/1 -> "FC ON?, EOem, MFex, Tex, O2ex"/1
  Integrator/1 -> cum fuel use (gal)/1
  [engine_on] -> "HOT engine maps "/Enable, Mux4/1, fc temp correct/Enable, fc temp/3(fc ON?)
  Selector3/1 -> fc temp correct/1(Coolant T (C)), To Workspace9/1, "HOT engine maps "/2(Coolant Temp), [coolant_temp]
  g/s-->gal/s/1 -> Integrator/1
  "HOT engine maps "/7(ex heat (W)) -> To Workspace12/1
  fc temp correct/2(EO emis (g/s)) -> Mux4/2, To Workspace8/1
  "HOT engine maps "/2(HOT fuel use (g/s)) -> fc temp correct/2(HOT fuel use (g/s))
  fc temp correct/1(fuel use (g/s)) -> System Efficiency/1(In1), To Workspace15/1, g/s-->gal/s/1
  "HOT engine maps "/6(O2 exhaust (g/s)) -> Mux4/5, To Workspace18/1

== system OUR_BD_FUELCELL/fuel cell control strategy <cs>/FC on/Subsystem ==
  in_1 : Inport
  Constant1 : Constant  Value=n
  Integrator : Integrator
  Product : Product  Inputs=*/  InputSameDT=on  RndMeth=Zero  SaturateOnIntegerOverflow=on  OutDataTypeStr=Inherit: Same as first input
  Sum : Sum  Inputs=+-  InputSameDT=on  SaturateOnIntegerOverflow=on  OutDataTypeStr=Inherit: Same as first input
  Transport Delay : TransportDelay  DelayTime=n
  out_1 : Outport  InitialOutput=0
  wires:
  Constant1/1 -> Product/2
  Product/1 -> out_1/1
  in_1/1 -> Integrator/1
  Sum/1 -> Product/1
  Transport Delay/1 -> Sum/2
  Integrator/1 -> Transport Delay/1, Sum/1

== system OUR_BD_FUELCELL/fuel cell control strategy <cs>/FC on/dt ==
  Clock : Clock
  Memory1 : Memory  InitialCondition=-1
  Sum1 : Sum  Inputs=+-  InputSameDT=on  SaturateOnIntegerOverflow=on  OutDataTypeStr=Inherit: Same as first input
  out_1 : Outport  InitialOutput=0
  wires:
  Sum1/1 -> out_1/1
  Memory1/1 -> Sum1/2
  Clock/1 -> Memory1/1, Sum1/1

== system OUR_BD_FUELCELL/fuel cell control strategy <cs>/FC on/just shut down ==
  state : Inport
  Logical Operator : Logic
  Logical Operator1 : Logic  Operator=NOT  Inputs=1
  Memory1 : Memory  InitialCondition=1
  trigger : Outport  InitialOutput=0
  wires:
  Logical Operator/1 -> trigger/1
  Memory1/1 -> Logical Operator/2
  state/1 -> Memory1/1, Logical Operator1/1
  Logical Operator1/1 -> Logical Operator/1

== system OUR_BD_FUELCELL/fuel cell control strategy <cs>/FC on/no-lag Reset Integrator ==
  in_1 : Inport
  in_2 : Inport  Port=2
  in_3 : Inport  Port=3
  Constant : Constant  Value=0
  Memory : Memory  InitialCondition=initval
  Product : Product  InputSameDT=on  RndMeth=Zero  SaturateOnIntegerOverflow=on  OutDataTypeStr=Inherit: Same as first input
  Sum : Sum  InputSameDT=on  SaturateOnIntegerOverflow=on  OutDataTypeStr=Inherit: Same as first input
  Switch : Switch  Threshold=eps
  dt : Subsystem
  in_2==0 : RelationalOperator  Operator===
  out_1 : Outport  InitialOutput=0
  wires:
  Constant/1 -> in_2==0/2
  in_2==0/1 -> Switch/2
  Switch/1 -> Memory/1, out_1/1
  Sum/1 -> Switch/1
  Memory/1 -> Sum/1
  Product/1 -> Sum/2
  dt/1(out_1) -> Product/1
  in_1/1 -> Product/2
  in_2/1 -> in_2==0/1
  in_3/1 -> Switch/3

== system OUR_BD_FUELCELL/fuel cell control strategy <cs>/FC on1/Subsystem ==
  in_1 : Inport
  Constant1 : Constant  Value=n
  Integrator : Integrator
  Product : Product  Inputs=*/  InputSameDT=on  RndMeth=Zero  SaturateOnIntegerOverflow=on  OutDataTypeStr=Inherit: Same as first input
  Sum : Sum  Inputs=+-  InputSameDT=on  SaturateOnIntegerOverflow=on  OutDataTypeStr=Inherit: Same as first input
  Transport Delay : TransportDelay  DelayTime=n
  out_1 : Outport  InitialOutput=0
  wires:
  Constant1/1 -> Product/2
  Product/1 -> out_1/1
  in_1/1 -> Integrator/1
  Sum/1 -> Product/1
  Transport Delay/1 -> Sum/2
  Integrator/1 -> Transport Delay/1, Sum/1

== system OUR_BD_FUELCELL/fuel cell control strategy <cs>/FC on1/dt ==
  Clock : Clock
  Memory1 : Memory  InitialCondition=-1
  Sum1 : Sum  Inputs=+-  InputSameDT=on  SaturateOnIntegerOverflow=on  OutDataTypeStr=Inherit: Same as first input
  out_1 : Outport  InitialOutput=0
  wires:
  Sum1/1 -> out_1/1
  Memory1/1 -> Sum1/2
  Clock/1 -> Memory1/1, Sum1/1

== system OUR_BD_FUELCELL/fuel cell control strategy <cs>/FC on1/just shut down ==
  state : Inport
  Logical Operator : Logic
  Logical Operator1 : Logic  Operator=NOT  Inputs=1
  Memory1 : Memory  InitialCondition=1
  trigger : Outport  InitialOutput=0
  wires:
  Logical Operator/1 -> trigger/1
  Memory1/1 -> Logical Operator/2
  state/1 -> Memory1/1, Logical Operator1/1
  Logical Operator1/1 -> Logical Operator/1

== system OUR_BD_FUELCELL/fuel cell control strategy <cs>/FC on1/no-lag Reset Integrator ==
  in_1 : Inport
  in_2 : Inport  Port=2
  in_3 : Inport  Port=3
  Constant : Constant  Value=0
  Memory : Memory  InitialCondition=initval
  Product : Product  InputSameDT=on  RndMeth=Zero  SaturateOnIntegerOverflow=on  OutDataTypeStr=Inherit: Same as first input
  Sum : Sum  InputSameDT=on  SaturateOnIntegerOverflow=on  OutDataTypeStr=Inherit: Same as first input
  Switch : Switch  Threshold=eps
  dt : Subsystem
  in_2==0 : RelationalOperator  Operator===
  out_1 : Outport  InitialOutput=0
  wires:
  Constant/1 -> in_2==0/2
  in_2==0/1 -> Switch/2
  Switch/1 -> Memory/1, out_1/1
  Sum/1 -> Switch/1
  Memory/1 -> Sum/1
  Product/1 -> Sum/2
  dt/1(out_1) -> Product/1
  in_1/1 -> Product/2
  in_2/1 -> in_2==0/1
  in_3/1 -> Switch/3

== system OUR_BD_FUELCELL/fuel cell control strategy <cs>/FC pwr command, modified by SOC/Block NOTES ==
  note: 1/5/98/98:tm  Modified calculation of additional power required to maintain goal SOC
      | (SOC_goal - SOC_actual) / (0.5*SOC_range) * cs_charge_pwr
      | therefore when
      | actual_SOC=cs_lo_soc ==> 1.0  *cs_charge_pwr
      | actual_SOC=goal_SOC ==> 0.0  *cs_charge_pwr
      | actual_SOC=cs_hi_soc ==> -1.0 * cs_charge_pwr
  note: This block determines the additional power required of the fuel convertor
      |  to maintian an SOC equal to the average of cs_hi_soc and cs_lo_soc.

== system OUR_BD_FUELCELL/fuel converter <fc> net model/fuel cell system <fc>/Block NOTES ==
  note: This block models the energy storage system as an SOC-dependent voltage
      | in series with an SOC- and current direction-dependent internal resistance.
      | SOC is computed assuming that A-h capacity is a function of average discharge
      | current:  (A-h capacity)=ess_peukert_coeff * (average discharge current)^ess_peukert_exp.
      |
      | Discharge power is limited here so as not to bring the bus (battery pack) voltage below
      | the minimum controller voltage and so as to allow the solution of the quadratic eq'n for
      | discharge current.
      |
      | Positive current is discharge current in the convention used here.
  note: Power loss is computed as I*R+losses due to Coulombic (in)efficiency.
  note: 7/30/98
      | - started with battery from BD_SER2h.m
      | - added a Saturation block to prevent computed
      |        SOC from falling below 0 or rising above 1
      | - added logic in 'limit power' to prevent discharge
      | if SOC is below 0.001 (0.1%)
      | -added limit block to check if low SOC is preventing
      | discharge

== system OUR_BD_FUELCELL/fuel converter <fc> net model/fuel cell system <fc>/pwr vs. eff fuel cell model ==
  net pwr req (W) : Inport
  Enable : EnablePort  StatesWhenEnabling=reset
  enforce limits : Subsystem
  net pwr avail (W) : Outport  OutputWhenDisabled=reset  InitialOutput=0
  wires:
  net pwr req (W)/1 -> enforce limits/1(In1)
  enforce limits/1(Out1) -> net pwr avail (W)/1

== system OUR_BD_FUELCELL/fuel converter <fc> net model/fuel use and EO emis Fuel Cell/Block NOTES ==
  note: This block determines actual fuel use and engine-out emissions
      | given the fully hot values and the engine coolant temperature.
      | The correlations used here were developed at NREL using
      | FTP data collected under subcontract by JDM & Associates.
      | Note: PM hot/cold relation assumed same as HC

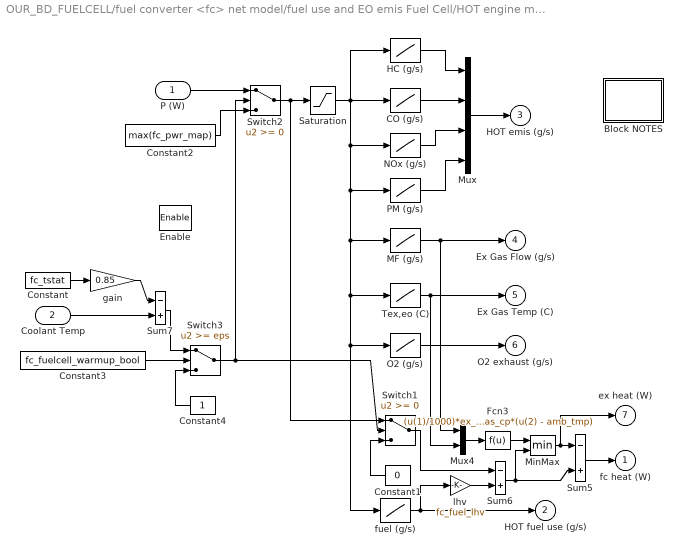
== system OUR_BD_FUELCELL/fuel converter <fc> net model/fuel use and EO emis Fuel Cell/HOT engine maps  ==
  P (W) : Inport
  Coolant Temp : Inport  Port=2
  Enable : EnablePort  StatesWhenEnabling=reset
  Block NOTES : Subsystem
      mask Display: disp('Block\nNOTES')
  CO (g/s) : Lookup  InputValues=fc_pwr_map*fc_pwr_scale  Table=fc_co_map*fc_pwr_scale
  Constant : Constant  Value=fc_tstat
  Constant1 : Constant  Value=0
  Constant2 : Constant  Value=max(fc_pwr_map)
  Constant3 : Constant  Value=fc_fuelcell_warmup_bool
  Constant4 : Constant
  Fcn3 : Fcn  Expr=(u(1)/1000)*ex_gas_cp*(u(2) - amb_tmp)
  HC (g/s) : Lookup  InputValues=fc_pwr_map*fc_pwr_scale  Table=fc_hc_map*fc_pwr_scale
  MF (g/s) : Lookup  InputValues=fc_pwr_map*fc_pwr_scale  Table=fc_exflow_map*fc_pwr_scale
  MinMax : MinMax  Inputs=2  InputSameDT=on  SaturateOnIntegerOverflow=on
  Mux : Mux
  Mux4 : Mux  Inputs=2
  NOx (g/s) : Lookup  InputValues=fc_pwr_map*fc_pwr_scale  Table=fc_nox_map*fc_pwr_scale
  O2 (g/s) : Lookup  InputValues=fc_pwr_map*fc_pwr_scale  Table=fc_o2_map*fc_pwr_scale
  PM (g/s) : Lookup  InputValues=fc_pwr_map*fc_pwr_scale  Table=fc_pm_map*fc_pwr_scale
  Saturation : Saturate  UpperLimit=max(fc_pwr_map*fc_pwr_scale)  LowerLimit=0
  Sum5 : Sum  Inputs=-+  InputSameDT=on  SaturateOnIntegerOverflow=on  OutDataTypeStr=Inherit: Same as first input
  Sum6 : Sum  Inputs=-+  InputSameDT=on  SaturateOnIntegerOverflow=on  OutDataTypeStr=Inherit: Same as first input
  Sum7 : Sum  Inputs=-+  InputSameDT=on  SaturateOnIntegerOverflow=on  OutDataTypeStr=Inherit: Same as first input
  Switch1 : Switch
  Switch2 : Switch
  Switch3 : Switch  Threshold=eps
  Tex,eo (C) : Lookup  InputValues=fc_pwr_map*fc_pwr_scale  Table=fc_extmp_map
  fuel (g/s) : Lookup  InputValues=fc_pwr_map*fc_pwr_scale  Table=fc_fuel_map*fc_pwr_scale/fc_eff_scale
  gain : Gain  Gain=0.85  SaturateOnIntegerOverflow=on  OutDataTypeStr=Inherit: Same as input  ParamDataTypeStr=Inherit: Same as input
  lhv : Gain  Gain=fc_fuel_lhv  SaturateOnIntegerOverflow=on  OutDataTypeStr=Inherit: Same as input  ParamDataTypeStr=Inherit: Same as input
  fc heat (W) : Outport  OutputWhenDisabled=reset  InitialOutput=eps
  HOT fuel use (g/s) : Outport  Port=2  OutputWhenDisabled=reset  InitialOutput=eps
  HOT emis (g/s) : Outport  Port=3  OutputWhenDisabled=reset  InitialOutput=eps
  Ex Gas Flow (g/s) : Outport  Port=4  OutputWhenDisabled=reset  InitialOutput=eps
  Ex Gas Temp (C) : Outport  Port=5  OutputWhenDisabled=reset  InitialOutput=amb_tmp
  O2 exhaust (g/s) : Outport  Port=6  OutputWhenDisabled=reset  InitialOutput=eps
  ex heat (W) : Outport  Port=7  OutputWhenDisabled=reset  InitialOutput=eps
  wires:
  Constant4/1 -> Switch3/3
  Constant/1 -> gain/1
  Coolant Temp/1 -> Sum7/2
  gain/1 -> Sum7/1
  Sum7/1 -> Switch3/1
  Constant3/1 -> Switch3/2
  Switch3/1 -> Switch2/2, Switch1/2
  Switch2/1 -> Switch1/1, Saturation/1
  Constant2/1 -> Switch2/3
  P (W)/1 -> Switch2/1
  PM (g/s)/1 -> Mux/4
  HC (g/s)/1 -> Mux/1
  NOx (g/s)/1 -> Mux/3
  Mux/1 -> HOT emis (g/s)/1
  MF (g/s)/1 -> Ex Gas Flow (g/s)/1, Mux4/1
  Tex,eo (C)/1 -> Ex Gas Temp (C)/1, Mux4/2
  Saturation/1 -> CO (g/s)/1, MF (g/s)/1, Tex,eo (C)/1, fuel (g/s)/1, O2 (g/s)/1, PM (g/s)/1, NOx (g/s)/1, HC (g/s)/1
  CO (g/s)/1 -> Mux/2
  Switch1/1 -> Sum6/1
  Mux4/1 -> Fcn3/1
  Sum5/1 -> fc heat (W)/1
  Fcn3/1 -> MinMax/1
  MinMax/1 -> Sum5/1, ex heat (W)/1
  Sum6/1 -> Sum5/2, MinMax/2
  lhv/1 -> Sum6/2
  Constant1/1 -> Switch1/3
  fuel (g/s)/1 -> HOT fuel use (g/s)/1, lhv/1
  O2 (g/s)/1 -> O2 exhaust (g/s)/1

== system OUR_BD_FUELCELL/fuel converter <fc> net model/fuel use and EO emis Fuel Cell/System Efficiency ==
  In1 : Inport
  Constant : Constant  Value=eps
  Gain : Gain  Gain=fc_fuel_lhv  SaturateOnIntegerOverflow=on  OutDataTypeStr=Inherit: Same as input  ParamDataTypeStr=Inherit: Same as input
  Gain1 : Gain  Gain=100  SaturateOnIntegerOverflow=on  OutDataTypeStr=Inherit: Same as input  ParamDataTypeStr=Inherit: Same as input
  Product : Product  Inputs=*/  InputSameDT=on  RndMeth=Zero  SaturateOnIntegerOverflow=on  OutDataTypeStr=Inherit: Same as first input
  Sum1 : Sum  Inputs=|++  InputSameDT=on  SaturateOnIntegerOverflow=on  OutDataTypeStr=Inherit: Same as first input
  To Workspace1 : ToWorkspace  VariableName=fc_eff_out_a  SampleTime=-1
  tag scope: fc_eff_out_a=global
  wires:
  In1/1 -> Gain/1
  Gain1/1 -> [fc_eff_out_a], To Workspace1/1
  Sum1/1 -> Product/2
  Constant/1 -> Sum1/2
  Gain/1 -> Sum1/1
  Product/1 -> Gain1/1
  [fc_pwr_out_a] -> Product/1

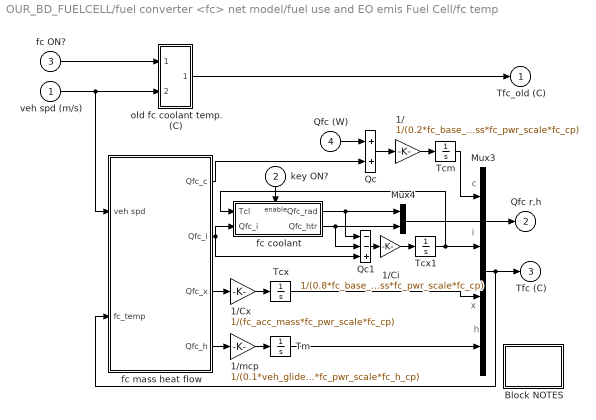
== system OUR_BD_FUELCELL/fuel converter <fc> net model/fuel use and EO emis Fuel Cell/fc temp ==
  note: h
  note: x
  note: i
  note: c
  veh spd (m/s) : Inport
  key ON? : Inport  Port=2
  fc ON? : Inport  Port=3
  Qfc (W) : Inport  Port=4
  "1/ " : Gain  Gain=1/(0.2*fc_base_mass*fc_pwr_scale*fc_cp)  SaturateOnIntegerOverflow=on  OutDataTypeStr=Inherit: Same as input  ParamDataTypeStr=Inherit: Same as input
  1/Ci : Gain  Gain=1/(0.8*fc_base_mass*fc_pwr_scale*fc_cp)  SaturateOnIntegerOverflow=on  OutDataTypeStr=Inherit: Same as input  ParamDataTypeStr=Inherit: Same as input
  1/Cx : Gain  Gain=1/(fc_acc_mass*fc_pwr_scale*fc_cp)  SaturateOnIntegerOverflow=on  OutDataTypeStr=Inherit: Same as input  ParamDataTypeStr=Inherit: Same as input
  1/mcp : Gain  Gain=1/(0.1*veh_glider_mass*fc_pwr_scale*fc_h_cp)  SaturateOnIntegerOverflow=on  OutDataTypeStr=Inherit: Same as input  ParamDataTypeStr=Inherit: Same as input
  Block NOTES : Subsystem
      mask Display: disp('Block\nNOTES')
  Mux3 : Mux
  Mux4 : Mux  Inputs=2
  Qc : Sum  InputSameDT=on  SaturateOnIntegerOverflow=on  OutDataTypeStr=Inherit: Same as first input
  Qc1 : Sum  Inputs=--+  InputSameDT=on  SaturateOnIntegerOverflow=on  OutDataTypeStr=Inherit: Same as first input
  Tcm : Integrator  InitialCondition=fc_c_init_tmp
  Tcx : Integrator  InitialCondition=fc_x_init_tmp
  Tcx1 : Integrator  InitialCondition=fc_i_init_tmp
  Tm : Integrator  InitialCondition=fc_h_init_tmp
  fc coolant : Subsystem  TreatAsAtomicUnit=on
  fc mass heat flow : Subsystem
  old fc coolant temp. (C) : Subsystem
  Tfc_old (C) : Outport  InitialOutput=0
  Qfc r,h : Outport  Port=2  InitialOutput=0
  Tfc (C) : Outport  Port=3  InitialOutput=0
  wires:
  Qc/1 -> "1/ "/1
  "1/ "/1 -> Tcm/1
  Qfc (W)/1 -> Qc/1
  fc mass heat flow/1(Qfc_c) -> Qc/2
  Qc1/1 -> 1/Ci/1
  1/Ci/1 -> Tcx1/1
  Tcm/1 -> Mux3/1
  fc mass heat flow/2(Qfc_i) -> Qc1/3, fc coolant/2("Qfc_i ")
  fc coolant/2(Qfc_htr) -> Qc1/2, Mux4/2
  fc coolant/1(Qfc_rad) -> Qc1/1, Mux4/1
  Tcx1/1 -> fc coolant/1(Tcl), Mux3/2
  Mux4/1 -> Qfc r,h/1
  1/Cx/1 -> Tcx/1
  fc mass heat flow/3(Qfc_x) -> 1/Cx/1
  key ON?/1 -> fc coolant/Enable
  Tcx/1 -> Mux3/3
  Tm/1 -> Mux3/4
  1/mcp/1 -> Tm/1
  fc mass heat flow/4(Qfc_h) -> 1/mcp/1
  Mux3/1 -> fc mass heat flow/2(fc_temp), Tfc (C)/1
  old fc coolant temp. (C)/1(fc coolant temp (C)) -> Tfc_old (C)/1
  veh spd (m/s)/1 -> old fc coolant temp. (C)/2(veh spd), fc mass heat flow/1(veh spd)
  fc ON?/1 -> old fc coolant temp. (C)/1(fc on?)
